simulink model "tf_to_c_sim"  (R2024b)
settings: Solver=FixedStepDiscrete  StartTime=0.0  StopTime=10.0  RelTol=1e-3
values from neighbouring files (symbols this model uses):
  input_values = single(reshape(input(index,:), [dim_1, dim_2]))    [tf_to_c_mat.m]
  temp_max = 184.88    [tf_to_c_mat.m]
  temp_min = 19.6    [tf_to_c_mat.m]
libraries: deeplib x1
settings Model: Creator=dx5entre  LastModifiedBy=dx5entre
settings OptimizationCC: DefaultParameterBehavior=Inlined  UseDivisionForNetSlopeComputation=on  GainParamInheritBuiltInType=on  UseFloatMulNetSlope=on  InlineInvariantSignals=on  PassReuseOutputArgsAs=Individual arguments  ZeroExternalMemoryAtStartup=off  ZeroInternalMemoryAtStartup=off  NoFixptDivByZeroProtection=on  EfficientFloat2IntCast=on  LifeSpan=1  OptimizeBlockOrder=speed  DifferentSizesBufferReuse=on  EfficientTunableParamExpr=on
settings DebuggingCC: ParameterTunabilityLossMsg=error
settings HardwareCC: ProdBitPerPointer=32  ProdBitPerSizeT=32  ProdBitPerPtrDiffT=32  ProdLargestAtomicInteger=Long  ProdLargestAtomicFloat=Double  ProdWordSize=32  ProdLongLongMode=on  ProdHWDeviceType=ARM Compatible->ARM Cortex-M
settings SFSimCC: MATLABDynamicMemAlloc=off
settings RTWCC: Description=Embedded Coder  SystemTargetFile=ert.tlc  TemplateMakefile=ert_default_tmf
settings CodeAppCC: ForceParamTrailComments=on  IgnoreCustomStorageClasses=off  OperatorAnnotations=on  SimulinkDataObjDesc=on  SFDataObjDesc=on  CustomSymbolStrGlobalVar=rt$N$M  CustomSymbolStrType=$N$M  CustomSymbolStrFcn=$N$M$F  CustomSymbolStrMacro=$N$M  InsertBlockDesc=on
settings ERTTargetCC: TargetLangStandard=C99 (ISO)  GenerateSampleERTMain=on  IncludeMdlTerminateFcn=off  CombineSignalStateStructs=on  SupportAbsoluteTime=off  SupportComplex=off  SupportNonInlinedSFcns=on  ERTCustomFileTemplate=example_file_process.tlc  ERTFilePackagingFormat=CompactWithDataFile

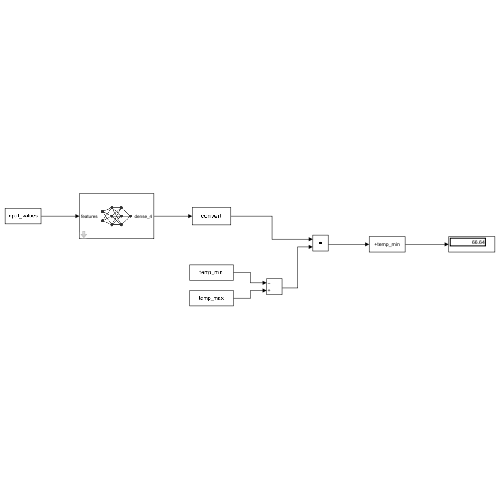
[thumbnail: Simulink's stored preview of the top-level diagram]
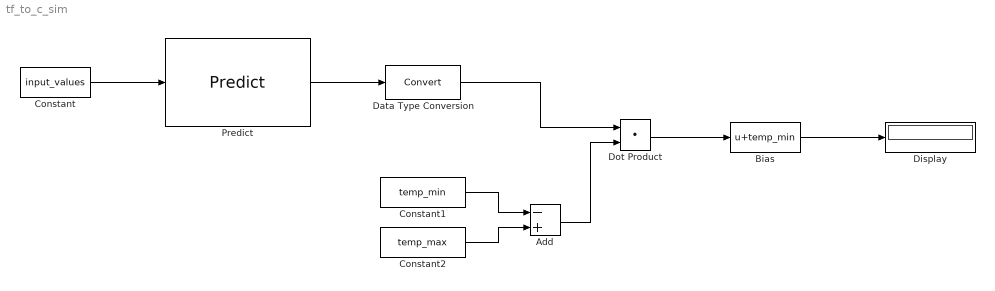
== system tf_to_c_sim ==
  Add : Sum  Inputs=-+
  Bias : Bias  Bias=temp_min  SaturateOnIntegerOverflow=off
  Constant : Constant  Value=input_values  VectorParams1D=off
  Constant1 : Constant  Value=temp_min
  Constant2 : Constant  Value=temp_max
  Data Type Conversion : DataTypeConversion  SaturateOnIntegerOverflow=off  RndMeth=Floor
  Display : Display
  Dot Product : DotProduct  OutDataTypeStr=Inherit: Inherit via internal rule
  Predict : deeplib/Predict  Network=Network from MAT-file  NetworkFunction=squeezenet  NetworkFilePath=C:\Users\dx5entre\Documents\Spang\edge-ai\Jupyter\models\Model_113_FCNN\Model_113_FCNN.mat  MiniBatchSize=128  InputDataFormats={ 'features', 'BC' }  Predictions=on  Activations={}  ForceInterpretedSim=off  EnableDLNetwork=on  LastKnownNetworkFilePath='C:\Users\dx5entre\Documents\Spang\edge-ai\Jupyter\models\Model_113_FCNN\Model_113_FCNN.mat'  LastKnownNetworkTimeStamp=739814.35143518517725169658660888671875
  wires:
  Constant2/1 -> Add/2
  Constant1/1 -> Add/1
  Add/1 -> Dot Product/2
  Dot Product/1 -> Bias/1
  Bias/1 -> Display/1
  Constant/1 -> Predict/1
  Data Type Conversion/1 -> Dot Product/1
  Predict/1 -> Data Type Conversion/1
